simulink model "thrirteenlevelinverter"  (R2013a)
settings: Solver=ode45  StartTime=0.0  StopTime=0.5  RelTol=1e-3
libraries: powerlib x22
settings Model: Creator=Dharma  LastModifiedBy=SRIDHARAN
settings DataIOCC: SignalLoggingSaveFormat=ModelDataLogs
settings OptimizationCC: ExpressionDepthLimit=2147483647
settings DebuggingCC: FcnCallInpInsideContextMsg=UseLocalSettings
settings GRTTargetCC: CombineOutputUpdateFcns=off  GRTInterface=on

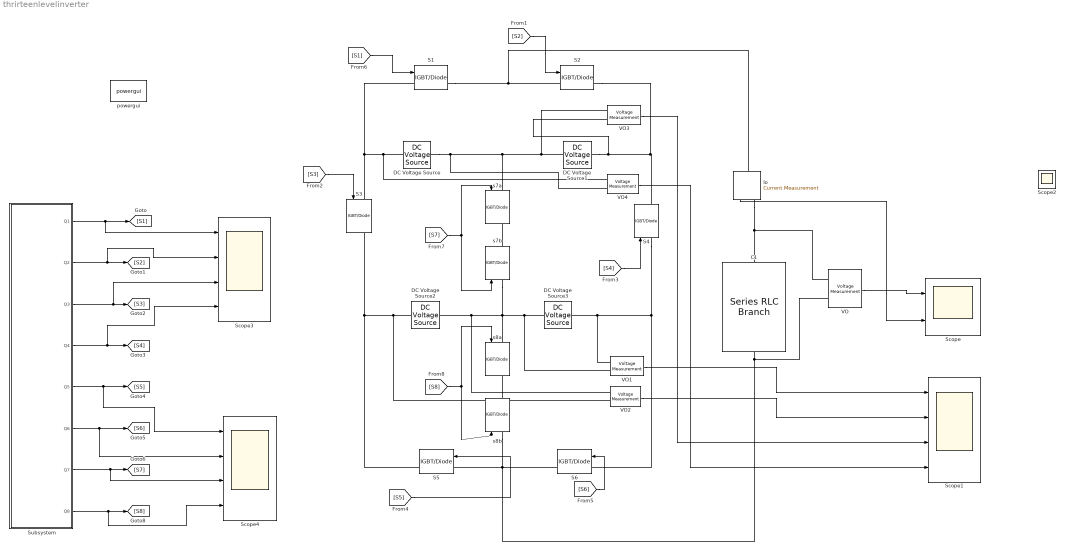
== system thrirteenlevelinverter ==
  C1 : powerlib/Elements/Series RLC Branch  LConnTagsString=__new0  RConnTagsString=__new0  BranchType=R  Resistance=47  Inductance=59e-3  SetiL0=off  InitialCurrent=0  Capacitance=2200e-6  Setx0=off  InitialVoltage=0  Measurements=None
  DC Voltage Source : powerlib/Electrical Sources/DC Voltage Source  Amplitude=100  Measurements=None
  DC Voltage Source1 : powerlib/Electrical Sources/DC Voltage Source  Amplitude=100  Measurements=None
  DC Voltage Source2 : powerlib/Electrical Sources/DC Voltage Source  Amplitude=50  Measurements=None
  DC Voltage Source3 : powerlib/Electrical Sources/DC Voltage Source  Amplitude=50  Measurements=None
  Io : powerlib/Measurements/Current Measurement  PhasorSimulation=off  OutputType=Complex  PSBequivalent=0
  S{1..6} (6 alike) : powerlib/Power Electronics/IGBT//Diode  Ron=1e-3  Rs=1e5  Cs=inf  Measurements=on
  Scope : Scope  NumInputPorts=2
      settings: YMin=-300~-5.5  YMax=300~5.5  SaveName=thd
  Scope1 : Scope  NumInputPorts=4
      settings: YMin=-225~-5~-5~-5  YMax=225~5~5~5  SaveName=thd1
  Scope2 : Scope
      settings: YMin=-225  YMax=225  SaveName=thd2
  Scope3 : Scope  NumInputPorts=4
      settings: YMin=-225~-5~-5~-5  YMax=225~5~5~5  SaveName=thd3
  Scope4 : Scope  NumInputPorts=4
      settings: YMin=-225~-5~-5~-5  YMax=225~5~5~5  SaveName=thd4
  Subsystem : Subsystem  mask{freq=50}
      mask prompts: freq "frequency"
  VO{,1..4} (5 alike) : powerlib/Measurements/Voltage Measurement  PhasorSimulation=off  OutputType=Complex  PSBequivalent=0
  powergui : powerlib/powergui  Priority=1  SimulationMode=Discrete  SolverType=Tustin  SampleTime=1e-6  frequency=60  SPID=off  DisableSnubberDevices=off  DisableRonSwitches=off  DisableVfSwitches=off  SwTol=0  Interpol=off  DisplayEquations=off  frequencyindice=0  Pbase=100e6  ErrMax=1e-4  Iterations=50  UnitsV=kV  UnitsW=MW  FunctionMessages=off  echomessages=off  HookPort=off  EnableUseOfTLC=off  x0status=blocks  RestoreLinks=warning  ResistiveCurrentMeasurement=off  Frange=[0:2:500]  Ylog=off  Xlog=on  ShowGrid=off  save=off  variable=ZData  structure=thd  ZoomFFT=off  StartTime=0.4  cycles=6  DisplayStyle=1  fundamental=50  FreqAxis=on  MaxFrequency=1000  frequencyindicesteady=1  RmsSteady=1  display=off  Ts=0  methode=off
  s7a : powerlib/Power Electronics/IGBT//Diode  Ron=1e-3  Rs=1e5  Cs=inf  Measurements=on
  s7b : powerlib/Power Electronics/IGBT//Diode  Ron=1e-3  Rs=1e5  Cs=inf  Measurements=on
  s8a : powerlib/Power Electronics/IGBT//Diode  Ron=1e-3  Rs=1e5  Cs=inf  Measurements=on
  s8b : powerlib/Power Electronics/IGBT//Diode  Ron=1e-3  Rs=1e5  Cs=inf  Measurements=on
  wires:
  VO/1 -> Scope/1
  Subsystem/1(Q1) -> Scope3/1, [S1]
  Subsystem/2(Q2) -> Scope3/2, [S2]
  Subsystem/3(Q3) -> Scope3/3, [S3]
  Subsystem/4(Q4) -> Scope3/4, [S4]
  Subsystem/5(Q5) -> Scope4/1, [S5]
  Subsystem/6(Q6) -> Scope4/2, [S6]
  Subsystem/7(Q7) -> Scope4/3, [S7]
  Subsystem/8(Q8) -> Scope4/4, [S8]
  [S1] -> S1/1
  [S2] -> S2/1
  [S3] -> S3/1
  [S4] -> S4/1
  [S5] -> S5/1
  [S6] -> S6/1
  [S7] -> s7a/1, s7b/1
  [S8] -> s8b/1, s8a/1
  Io/1 -> Scope/2
  VO1/1 -> Scope1/1
  VO2/1 -> Scope1/2
  VO4/1 -> Scope1/4
  VO3/1 -> Scope1/3
  connections:
  s7b/RConn1 -- s7a/RConn1
  DC Voltage Source/LConn1 -- VO4/LConn2 -- VO3/LConn1 -- DC Voltage Source1/RConn1 -- s7a/LConn1
  S3/LConn1 -- S1/LConn1 -- VO4/LConn1 -- DC Voltage Source/RConn1
  DC Voltage Source2/LConn1 -- VO2/LConn2 -- S3/RConn1 -- S5/RConn1
  s7b/LConn1 -- s8a/LConn1 -- DC Voltage Source3/LConn1 -- VO1/LConn2 -- VO2/LConn1 -- DC Voltage Source2/RConn1
  DC Voltage Source1/LConn1 -- VO3/LConn2 -- S2/RConn1 -- S4/RConn1
  S4/LConn1 -- S6/LConn1 -- VO1/LConn1 -- DC Voltage Source3/RConn1
  s8b/RConn1 -- s8a/RConn1
  s8b/LConn1 -- C1/RConn1 -- VO/LConn2 -- S6/RConn1 -- S5/LConn1
  S1/RConn1 -- Io/LConn1 -- S2/LConn1
  Io/RConn1 -- VO/LConn1 -- C1/LConn1

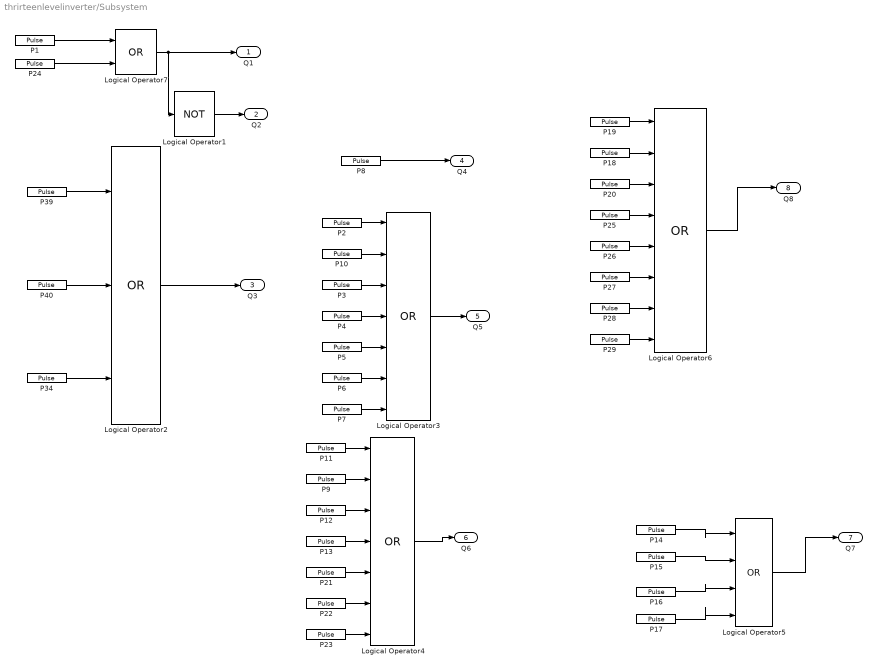
== system thrirteenlevelinverter/Subsystem ==
  Logical Operator1 : Logic  Operator=NOT  IconShape=distinctive  AllPortsSameDT=off  OutDataTypeStr=boolean
  Logical Operator2 : Logic  Operator=OR  Inputs=3  IconShape=distinctive  AllPortsSameDT=off  OutDataTypeStr=boolean
  Logical Operator3 : Logic  Operator=OR  Inputs=7  IconShape=distinctive  AllPortsSameDT=off  OutDataTypeStr=boolean
  Logical Operator4 : Logic  Operator=OR  Inputs=7  IconShape=distinctive  AllPortsSameDT=off  OutDataTypeStr=boolean
  Logical Operator5 : Logic  Operator=OR  Inputs=4  IconShape=distinctive  AllPortsSameDT=off  OutDataTypeStr=boolean
  Logical Operator6 : Logic  Operator=OR  Inputs=8  IconShape=distinctive  AllPortsSameDT=off  OutDataTypeStr=boolean
  Logical Operator7 : Logic  Operator=OR  IconShape=distinctive  AllPortsSameDT=off  OutDataTypeStr=boolean
  P1 : DiscretePulseGenerator  PulseType=Time based  Period=1/freq  PulseWidth=(100/24)*12
  P10 : DiscretePulseGenerator  PulseType=Time based  Period=1/freq  PulseWidth=(100/24)  PhaseDelay=((1/freq)/24)*5
  P11 : DiscretePulseGenerator  PulseType=Time based  Period=1/freq  PulseWidth=(100/24)
  P12 : DiscretePulseGenerator  PulseType=Time based  Period=1/freq  PulseWidth=(100/24)  PhaseDelay=((1/freq)/24)*7
  P13 : DiscretePulseGenerator  PulseType=Time based  Period=1/freq  PulseWidth=(100/24)  PhaseDelay=((1/freq)/24)*10
  P14 : DiscretePulseGenerator  PulseType=Time based  Period=1/freq  PulseWidth=(100/24)*3
  P15 : DiscretePulseGenerator  PulseType=Time based  Period=1/freq  PulseWidth=(100/24)*3  PhaseDelay=((1/freq)/24)*8
  P16 : DiscretePulseGenerator  PulseType=Time based  Period=1/freq  PulseWidth=(100/24)*3  PhaseDelay=((1/freq)/24)*12
  P17 : DiscretePulseGenerator  PulseType=Time based  Period=1/freq  PulseWidth=(100/24)*3  PhaseDelay=((1/freq)/24)*19
  P18 : DiscretePulseGenerator  PulseType=Time based  Period=1/freq  PulseWidth=(100/24)  PhaseDelay=((1/freq)/24)*4
  P19 : DiscretePulseGenerator  PulseType=Time based  Period=1/freq  PulseWidth=(100/24)  PhaseDelay=((1/freq)/24)
  P2 : DiscretePulseGenerator  PulseType=Time based  Period=1/freq  PulseWidth=(100/24)  PhaseDelay=((1/freq)/24)*2
  P20 : DiscretePulseGenerator  PulseType=Time based  Period=1/freq  PulseWidth=(100/24)  PhaseDelay=((1/freq)/24)*6
  P21 : DiscretePulseGenerator  PulseType=Time based  Period=1/freq  PulseWidth=(100/24)  PhaseDelay=((1/freq)/24)*14
  P22 : DiscretePulseGenerator  PulseType=Time based  Period=1/freq  PulseWidth=(100/24)  PhaseDelay=((1/freq)/24)*17
  P23 : DiscretePulseGenerator  PulseType=Time based  Period=1/freq  PulseWidth=(100/24)  PhaseDelay=((1/freq)/24)*20
  P24 : DiscretePulseGenerator  PulseType=Time based  Period=1/freq  PulseWidth=(100/24)  PhaseDelay=((1/freq)/24)*23
  P25 : DiscretePulseGenerator  PulseType=Time based  Period=1/freq  PulseWidth=(100/24)  PhaseDelay=((1/freq)/24)*9
  P26 : DiscretePulseGenerator  PulseType=Time based  Period=1/freq  PulseWidth=(100/24)  PhaseDelay=((1/freq)/24)*13
  P27 : DiscretePulseGenerator  PulseType=Time based  Period=1/freq  PulseWidth=(100/24)  PhaseDelay=((1/freq)/24)*16
  P28 : DiscretePulseGenerator  PulseType=Time based  Period=1/freq  PulseWidth=(100/24)  PhaseDelay=((1/freq)/24)*18
  P29 : DiscretePulseGenerator  PulseType=Time based  Period=1/freq  PulseWidth=(100/24)  PhaseDelay=((1/freq)/24)*21
  P3 : DiscretePulseGenerator  PulseType=Time based  Period=1/freq  PulseWidth=(100/24)  PhaseDelay=((1/freq)/24)*8
  P34 : DiscretePulseGenerator  PulseType=Time based  Period=1/freq  PulseWidth=(100/24)  PhaseDelay=((1/freq)/24)*23
  P39 : DiscretePulseGenerator  PulseType=Time based  Period=1/freq  PulseWidth=(100/24)  PhaseDelay=((1/freq)/24)*11
  P4 : DiscretePulseGenerator  PulseType=Time based  Period=1/freq  PulseWidth=(100/24)*2  PhaseDelay=((1/freq)/24)*11
  P40 : DiscretePulseGenerator  PulseType=Time based  Period=1/freq  PulseWidth=(100/24)*5  PhaseDelay=((1/freq)/24)*15
  P5 : DiscretePulseGenerator  PulseType=Time based  Period=1/freq  PulseWidth=(100/24)  PhaseDelay=((1/freq)/24)*15
  P6 : DiscretePulseGenerator  PulseType=Time based  Period=1/freq  PulseWidth=(100/24)  PhaseDelay=((1/freq)/24)*19
  P7 : DiscretePulseGenerator  PulseType=Time based  Period=1/freq  PulseWidth=(100/24)*2  PhaseDelay=((1/freq)/24)*22
  P8 : DiscretePulseGenerator  PulseType=Time based  Period=1/freq  PulseWidth=(100/24)*5  PhaseDelay=((1/freq)/24)*3
  P9 : DiscretePulseGenerator  PulseType=Time based  Period=1/freq  PulseWidth=(100/24)  PhaseDelay=((1/freq)/24)*3
  Q1 : Outport
  Q2 : Outport  Port=2
  Q3 : Outport  Port=3
  Q4 : Outport  Port=4
  Q5 : Outport  Port=5
  Q6 : Outport  Port=6
  Q7 : Outport  Port=7
  Q8 : Outport  Port=8
  wires:
  P8/1 -> Q4/1
  Logical Operator7/1 -> Logical Operator1/1, Q1/1
  P1/1 -> Logical Operator7/1
  P24/1 -> Logical Operator7/2
  Logical Operator2/1 -> Q3/1
  P40/1 -> Logical Operator2/2
  P39/1 -> Logical Operator2/1
  P34/1 -> Logical Operator2/3
  Logical Operator3/1 -> Q5/1
  P2/1 -> Logical Operator3/1
  P10/1 -> Logical Operator3/2
  P15/1 -> Logical Operator5/2
  P14/1 -> Logical Operator5/1
  P16/1 -> Logical Operator5/3
  P17/1 -> Logical Operator5/4
  Logical Operator5/1 -> Q7/1
  Logical Operator1/1 -> Q2/1
  P3/1 -> Logical Operator3/3
  P4/1 -> Logical Operator3/4
  P5/1 -> Logical Operator3/5
  P6/1 -> Logical Operator3/6
  P7/1 -> Logical Operator3/7
  P11/1 -> Logical Operator4/1
  P9/1 -> Logical Operator4/2
  P12/1 -> Logical Operator4/3
  P13/1 -> Logical Operator4/4
  P21/1 -> Logical Operator4/5
  P22/1 -> Logical Operator4/6
  P23/1 -> Logical Operator4/7
  Logical Operator4/1 -> Q6/1
  P19/1 -> Logical Operator6/1
  P18/1 -> Logical Operator6/2
  P20/1 -> Logical Operator6/3
  P25/1 -> Logical Operator6/4
  P26/1 -> Logical Operator6/5
  P27/1 -> Logical Operator6/6
  P28/1 -> Logical Operator6/7
  Logical Operator6/1 -> Q8/1
  P29/1 -> Logical Operator6/8
